simulink model "DR18E_Testpult"  (R2017a)
settings: Solver=ode1  StartTime=0.0  StopTime=Inf  FixedStep=0.001  RelTol=1e-3
PostLoadFcn:
  | , if any(exist('dsrtsu_mdlpostloadfcn', 'file') == [2, 3, 6]), try dsrtsu_mdlpostloadfcn('Execute', bdroot); catch fprintf('Error in PostLoadFcn (dsrtsu_mdlpostloadfcn) for model "%s":\n %s\n', bdroot, lasterr); end, end,
model workspace: external: MATLAB File C:\Users\DeltaRacing\Documents\dSPACE\MABX_DR18E\Model\DR18E_MABX_Parameter.m (data not in the file)
values from neighbouring files (symbols this model uses):
  am = 1/Ts    (= 1)    [DR18E_MABX_Parameter.m]
  bm = K/Ts    (= 0.05)    [DR18E_MABX_Parameter.m]
  cf = 41350    [DR18E_MABX_Parameter.m]
  cr = 41350    [DR18E_MABX_Parameter.m]
  Derating_HV_Battery_Kapa = 1    [DR18E_MABX_Parameter.m]
  Derating_Start_km = 16    [DR18E_MABX_Parameter.m]
  Drive_Mode = 0    [DR18E_MABX_Parameter.m]
  g = 1    [DR18E_MABX_Parameter.m]
  Gas_Modus = 2    [DR18E_MABX_Parameter.m]
  HV_Power_max = 80    [DR18E_MABX_Parameter.m]
  i_Getriebe = 3.3    [DR18E_MABX_Parameter.m]
  i_Lenkgetriebe = 4.32    [DR18E_MABX_Parameter.m]
  K_SET = 1    [DR18E_MABX_Parameter.m]
  Kapazitaet_HV_Battery_kWh = 6.6    [DR18E_MABX_Parameter.m]
  KW_T_Soll = 37    [DR18E_MABX_Parameter.m]
  lf = 1.2    [DR18E_MABX_Parameter.m]
  lr = 1.15    [DR18E_MABX_Parameter.m]
  m = 310    [DR18E_MABX_Parameter.m]
  M_max = 150    [DR18E_MABX_Parameter.m]
  Power_Limit_onoff = 0    [DR18E_MABX_Parameter.m]
  Reifenradius = 0.2351    [DR18E_MABX_Parameter.m]
  Strecke_Endu_km = 22    [DR18E_MABX_Parameter.m]
  TC_Decr_Gas = 0.00005    (= 5e-05)    [DR18E_MABX_Parameter.m]
  TC_Derivative = 0.4    [DR18E_MABX_Parameter.m]
  TC_Incr_Gas = 0.005    [DR18E_MABX_Parameter.m]
  TC_On = 0    [DR18E_MABX_Parameter.m]
  TC_Relay_Off = 0.065    [DR18E_MABX_Parameter.m]
  TC_Relay_On = 0.07    [DR18E_MABX_Parameter.m]
  TV_Mode = 2    [DR18E_MABX_Parameter.m]
  TV_On = 0    [DR18E_MABX_Parameter.m]
  TV_Override = 1    [DR18E_MABX_Parameter.m]
  y = 0.8    [DR18E_MABX_Parameter.m]
undefined symbols (not defined in the file or in its folder): D, DiscIntNeverNeededParam, I, K_OL, P
libraries: simulink x288, rtican x105, rtiusbflightreclib x40, rti1401lib_dio_type3 x10, simulink_extras x10, rti1401lib_adc_type4 x8, rti1401lib_II_base x7
(part 18 of 28)

== system DR18E_Testpult/Verarbeitung/DR18E Torque Control/Derating ==
  note: wenn deltaStrecke
      | > 0 kein Derating
      | < 0 Derating
  In1 : Inport
  0-1 : Saturate  UpperLimit=1  LowerLimit=0
  0-80 : Saturate  UpperLimit=80  LowerLimit=0
  Bus Selector : BusSelector  OutputSignals=TagesenergieMABX_Wh,TagesmeterMABX_m
  Bus Selector1 : BusSelector  OutputSignals=TagesenergieMABX_Wh,TagesmeterMABX_m
  Constant2 : Constant  Value=HV_Power_max
  Derating_Strategie_Reichweite : Subsystem
  MinMax : MinMax  Inputs=2
  Product : Product
  PowerLimit_kW : Outport
  wires:
  In1/1 -> Bus Selector1/1, Bus Selector/1
  Bus Selector/1 -> Derating_Strategie_Reichweite/1(In1)  "<TagesenergieMABX_Wh>"
  Bus Selector/2 -> Derating_Strategie_Reichweite/2(In2)  "<TagesmeterMABX_m>"
  Derating_Strategie_Reichweite/1(deltaStrecke_km) -> MinMax/1
  MinMax/1 -> 0-1/1
  Constant2/1 -> 0-80/1
  Product/1 -> PowerLimit_kW/1
  0-1/1 -> Product/2
  0-80/1 -> Product/1

== system DR18E_Testpult/Verarbeitung/DR18E Torque Control/FlightRecorder ==
  In1 : Inport
  Data Type Conversion : DataTypeConversion
  Gain : Gain
  USB_FLIGHT_REC_BL1 : rtiusbflightreclib/USB_FLIGHT_REC_BL1  VarName=M_max_pro_Mot_Nm  DataType=Single  SampleTime=-1  TLCFileName=rtiusbflightrecwrite  Reserved1=[]  Reserved2=[]  Reserved3=[]  Reserved4=[]  DSProperties=struct('RTI',struct('Version',uint32(3),'BlockType',struct('isSLSource',uint8(0),'isSLSink',uint8(1),'isHWSource',uint8(0),'isHWSink',uint8(0),'isSetup',uint8(0),'isInline',uint8(1),'isNonInline',uint8(0),'isInterrupt',uint8(0),'isChannelwise',uint8(0)),'IOBoardType',{{'DSUSB','FLIGHTREC'}},'UnitType','FLIGHTREC','Identifier','WRITE','DialogType','SL','BlockSet','RTIUSBFLIGHTREC','SlaveProcessor','NONE'))  RTIBlockInterface=struct('InputPortsActive',1,'InputPortsWidth',int32(1),'InputPortsDataType',{{'SS_SINGLE'}},'BlockDisplay',{{['Write to\nUSB Flight Recorder'],'center'}},'IconTransparency','off','InitLevel',3,'BlockName',struct('Token',{{'USB_FLIGHT_REC_BL1'}}),'MaskDescription',['Write input to the Flight Recorder. Recorded data can be referenced by the specified variable.'],'SampleTime',{{-1}})  RTIBlockParameters=struct('VarName',{{'M_max_pro_Mot_Nm','OFF',[]}},'DataType',{{'Single','OFF',[]}},'SampleTime',{{-1,'OFF',[]}},'TLCFileName',{{'rtiusbflightrecwrite','OFF',[]}})  RTISFcnParameters=struct('VarName','char','DataType','char','SampleTime','double','TLCFileName','char')  RTIBlockParaDefault=struct('VarName','Var1','DataType','Single','SampleTime',-1,'TLCFileName','rtiusbflightrecwrite')
      settings: SourceProductName=dSPACE RTI USB Flight Rec Blockset
  wires:
  Gain/1 -> Data Type Conversion/1
  In1/1 -> Gain/1
  Data Type Conversion/1 -> USB_FLIGHT_REC_BL1/1

== system DR18E_Testpult/Verarbeitung/DR18E Torque Control/Power Limit ==
  note: M = P / (2*pi*n)
  note: Power Limit Calculation
  Power Limit onoff : Inport
  DriverTorqueRequest L [Nm] : Inport  Port=2
  DriverTorqueRequest R [Nm] : Inport  Port=3
  Inputs : Inport  Port=4
  Power Limit kW : Inport  Port=5
  Bus Selector : BusSelector  OutputSignals=HV_Power_Watt,Bus.Drehzahl_RL_rad/s,Bus.Drehzahl_RR_rad/s
  Demux : Demux  Outputs=2
  Divide : Product  Inputs=*/
  Divide1 : Product  Inputs=*/
  Divide2 : Product  Inputs=*/
  Logical Operator : Logic  Operator=NOT  AllPortsSameDT=off  OutDataTypeStr=boolean
  Logical Operator1 : Logic  Operator=OR  AllPortsSameDT=off  OutDataTypeStr=boolean
  Mux : Mux  Inputs=2
  Mux1 : Mux  Inputs=2
  Power Limit truefalse : RelationalOperator  Operator=<=  RndMeth=Nearest
  PowerLimit [kW]2 : Constant  Value=0.1
  Product : Product
  RPM-1/s : Gain  Gain=2*pi/(60)
  RPM-1/s1 : Gain  Gain=2*pi/(60)
  Sum1 : Sum  Inputs=-|+
  Sum2 : Sum  Inputs=|++
  Sum3 : Sum  Inputs=++|
  Sum5 : Sum  Inputs=++|
  Switch : Switch  Criteria=u2 > Threshold
  eps : Constant  Value=0.1
  halbe Gesamtleistung pro Motor : Gain  Gain=0.5
  kW-W : Gain  Gain=1000
  "rad/s -> RPM" : Gain  Gain=60/2*pi
  "rad/s -> RPM1" : Gain  Gain=60/2*pi
  LimitedTorque L [Nm] : Outport
  LimitedTorque R [Nm] : Outport  Port=2
  wires:
  Bus Selector/1 -> Power Limit truefalse/1  "<HV_Power_Watt>"
  Power Limit kW/1 -> kW-W/1
  DriverTorqueRequest L [Nm]/1 -> Divide/1, Mux/1
  DriverTorqueRequest R [Nm]/1 -> Sum5/1, Mux/2
  Demux/1 -> LimitedTorque L [Nm]/1
  Demux/2 -> LimitedTorque R [Nm]/1
  Divide/1 -> Product/1
  Product/1 -> Divide1/1, Sum1/1  "PMotL"
  halbe Gesamtleistung pro Motor/1 -> Product/2
  Mux1/1 -> Switch/3  "Torque_in_lim"
  Sum1/1 -> Divide2/1  "PMotR"
  Sum3/1 -> RPM-1/s1/1
  Sum2/1 -> RPM-1/s/1
  eps/1 -> Sum3/1, Sum2/2
  RPM-1/s/1 -> Divide1/2
  RPM-1/s1/1 -> Divide2/2
  Bus Selector/3 -> "rad/s -> RPM1"/1  "<Drehzahl_RR_rad/s>"
  "rad/s -> RPM"/1 -> Sum2/1
  "rad/s -> RPM1"/1 -> Sum3/2
  Divide2/1 -> Mux1/2  "MR"
  Divide1/1 -> Mux1/1  "ML"
  PowerLimit [kW]2/1 -> Sum5/2
  Sum5/1 -> Divide/2
  kW-W/1 -> Sum1/2, Power Limit truefalse/2, halbe Gesamtleistung pro Motor/1
  Power Limit truefalse/1 -> Logical Operator1/2  "Input_Threshold"
  Inputs/1 -> Bus Selector/1
  Bus Selector/2 -> "rad/s -> RPM"/1  "<Drehzahl_RL_rad/s>"
  Switch/1 -> Demux/1  "Torque_out"
  Mux/1 -> Switch/1  "Torque_in"
  Logical Operator/1 -> Logical Operator1/1
  Power Limit onoff/1 -> Logical Operator/1
  Logical Operator1/1 -> Switch/2  "Power Limit aktivnaktiv"

== system DR18E_Testpult/Verarbeitung/DR18E Torque Control/TC RL ==
  TC_On : Inport
  Gas_0-1 : Inport  Port=2
  Inputs : Inport  Port=3
  Bus Selector : BusSelector  OutputSignals=long_slip_left
  Switch : Switch  Criteria=u2 > Threshold
  Traction Control RL : Subsystem
  Logs : Outport
  Motor_Gas_RL : Outport  Port=2
  wires:
  Bus Selector/1 -> Traction Control RL/2(Car.LongSlip)  "<long_slip_left>"
  Gas_0-1/1 -> Switch/3, Traction Control RL/1(Gas_0-1)
  Switch/1 -> Motor_Gas_RL/1
  TC_On/1 -> Switch/2
  Traction Control RL/1(E_Gas) -> Logs/1, Switch/1  "E_Gas_RL"
  Inputs/1 -> Bus Selector/1

== system DR18E_Testpult/Verarbeitung/DR18E Torque Control/TC RR ==
  TC_On : Inport
  Gas_0-1 : Inport  Port=2
  Inputs : Inport  Port=3
  Bus Selector : BusSelector  OutputSignals=long_slip_right
  Switch : Switch  Criteria=u2 > Threshold
  Traction Control RR : Subsystem
  Logs : Outport
  Motor_Gas_RR : Outport  Port=2
  wires:
  Bus Selector/1 -> Traction Control RR/2(Car.LongSlip)  "<long_slip_right>"
  Gas_0-1/1 -> Switch/3, Traction Control RR/1(Gas_0-1)
  Switch/1 -> Motor_Gas_RR/1
  TC_On/1 -> Switch/2
  Traction Control RR/1(E_Gas) -> Logs/1, Switch/1  "E_Gas_RR"
  Inputs/1 -> Bus Selector/1

== system DR18E_Testpult/Verarbeitung/DR18E Torque Control/TV RL ==
  Inputs : Inport
  Bus Selector : BusSelector  OutputSignals=v_kmh,Bus.signal3.RX_Gyro_deg/s.Yaw_Z,Bus.signal3.RX_Lenkwinkel.Steering
  Bus Selector1 : BusSelector  OutputSignals=Bus.signal3.RX_Lenkwinkel.RX Timeout Error,Bus.signal3.RX_Gyro_deg/s.RX Timeout Error
  Constant1 : Constant  Value=0
  Constant2 : Constant  Value=TV_Mode
  Constant3 : Constant  Value=0
  Constant4 : Constant  Value=TV_On
  Gravity2 : Gain  Gain=K_SET
  Lenkwinkel-->Radeinschlagwinkel : Gain  Gain=1/i_Lenkgetriebe
  Logical Operator1 : Logic  AllPortsSameDT=off  OutDataTypeStr=boolean
  MRAC_PT1_Lyapunov : Subsystem
  MRAC_PT1_MIT_DIFF : Subsystem
  MRAC_PT1_MIT_NORM : Subsystem
  Multiport Switch TV : MultiPortSwitch  Inputs=5  DataPortForDefault=Additional data port
  Safety TV off : Logic  Operator=NOR  AllPortsSameDT=off  OutDataTypeStr=boolean
  Switch : Switch  Criteria=u2 > Threshold
  TV DR17E : Subsystem
  TV IPG : Subsystem
  "YawRate SET_NEW " : Subsystem
  deg-rad : Gain  Gain=2*pi/360
  deg-rad1 : Gain  Gain=2*pi/360
  kmh-ms : Gain  Gain=1/3.6
  TV RL Nm : Outport
  wires:
  Inputs/1 -> Bus Selector1/1, Bus Selector/1
  Gravity2/1 -> MRAC_PT1_Lyapunov/1(YawRate REF (rad/s)), MRAC_PT1_MIT_DIFF/1(YawRate REF (rad/s)), MRAC_PT1_MIT_NORM/1(YawRate REF (rad/s))
  "YawRate SET_NEW "/1(YawRate REF (rad/s)) -> Gravity2/1
  TV IPG/1(Out1) -> Multiport Switch TV/2
  MRAC_PT1_Lyapunov/1(Delta M (Nm)) -> Multiport Switch TV/3
  MRAC_PT1_MIT_NORM/1(Delta M (Nm)) -> Multiport Switch TV/4
  MRAC_PT1_MIT_DIFF/1(Delta M (Nm)) -> Multiport Switch TV/5
  Switch/1 -> TV RL Nm/1
  Multiport Switch TV/1 -> Switch/1  "Delta M Nm"
  Constant1/1 -> Switch/3
  Constant2/1 -> Multiport Switch TV/1
  Constant3/1 -> Multiport Switch TV/7
  Bus Selector1/1 -> Safety TV off/1  "<RX Timeout Error>"
  TV DR17E/1(Delta M (Nm)) -> Multiport Switch TV/6
  Constant4/1 -> Logical Operator1/1
  Logical Operator1/1 -> Switch/2
  Safety TV off/1 -> Logical Operator1/2
  Bus Selector/1 -> kmh-ms/1  "<v_kmh>"
  Bus Selector/2 -> TV DR17E/3(psipunkt_ist_deg_s), deg-rad/1  "<Yaw_Z>"
  deg-rad/1 -> MRAC_PT1_MIT_DIFF/2(Car.YawRate), MRAC_PT1_MIT_NORM/2(Car.YawRate), MRAC_PT1_Lyapunov/2(Car.YawRate), TV IPG/2(In3)
  Lenkwinkel-->Radeinschlagwinkel/1 -> TV DR17E/2(Radeinschlagwinkel_deg), deg-rad1/1
  kmh-ms/1 -> TV DR17E/1(vx_ms), "YawRate SET_NEW "/2(v_ms), TV IPG/1(In2)
  Bus Selector/3 -> Lenkwinkel-->Radeinschlagwinkel/1  "<Steering>"
  deg-rad1/1 -> "YawRate SET_NEW "/1(Radeinschlagwinkel_rad)
  Bus Selector1/2 -> Safety TV off/2  "<RX Timeout Error>"

== system DR18E_Testpult/Verarbeitung/DR18E Torque Control/TV RR ==
  Inputs : Inport
  Bus Selector : BusSelector  OutputSignals=v_kmh,Bus.signal3.RX_Gyro_deg/s.Yaw_Z,Bus.signal3.RX_Lenkwinkel.Steering
  Bus Selector1 : BusSelector  OutputSignals=Bus.signal3.RX_Gyro_deg/s.RX Timeout Error,Bus.signal3.RX_Lenkwinkel.RX Timeout Error
  Constant1 : Constant  Value=0
  Constant2 : Constant  Value=TV_Mode
  Constant3 : Constant  Value=0
  Constant4 : Constant  Value=TV_On
  Gravity2 : Gain  Gain=K_SET
  Lenkwinkel-->Radeinschlagwinkel : Gain  Gain=1/i_Lenkgetriebe
  Logical Operator1 : Logic  AllPortsSameDT=off  OutDataTypeStr=boolean
  MRAC_PT1_Lyapunov : Subsystem
  MRAC_PT1_MIT_DIFF : Subsystem
  MRAC_PT1_MIT_NORM : Subsystem
  Multiport Switch TV : MultiPortSwitch  Inputs=5  DataPortForDefault=Additional data port
  Safety TV off : Logic  Operator=NOR  AllPortsSameDT=off  OutDataTypeStr=boolean
  Switch : Switch  Criteria=u2 > Threshold
  TV DR17E : Subsystem
  TV IPG : Subsystem
  "YawRate SET_NEW " : Subsystem
  deg-rad : Gain  Gain=2*pi/360
  deg-rad1 : Gain  Gain=2*pi/360
  kmh-ms : Gain  Gain=1/3.6
  TV RR Nm : Outport
  wires:
  Inputs/1 -> Bus Selector1/1, Bus Selector/1
  Gravity2/1 -> MRAC_PT1_Lyapunov/1(YawRate REF (rad/s)), MRAC_PT1_MIT_DIFF/1(YawRate REF (rad/s)), MRAC_PT1_MIT_NORM/1(YawRate REF (rad/s))
  "YawRate SET_NEW "/1(YawRate REF (rad/s)) -> Gravity2/1
  TV IPG/1(Out1) -> Multiport Switch TV/2
  MRAC_PT1_Lyapunov/1(Delta M (Nm)) -> Multiport Switch TV/3
  MRAC_PT1_MIT_NORM/1(Delta M (Nm)) -> Multiport Switch TV/4
  MRAC_PT1_MIT_DIFF/1(Delta M (Nm)) -> Multiport Switch TV/5
  Switch/1 -> TV RR Nm/1
  Multiport Switch TV/1 -> Switch/1  "Delta M Nm"
  Constant1/1 -> Switch/3
  Constant2/1 -> Multiport Switch TV/1
  Constant3/1 -> Multiport Switch TV/7
  Bus Selector1/1 -> Safety TV off/1  "<RX Timeout Error>"
  TV DR17E/1(Delta M (Nm)) -> Multiport Switch TV/6
  Constant4/1 -> Logical Operator1/1
  Logical Operator1/1 -> Switch/2
  Safety TV off/1 -> Logical Operator1/2
  Bus Selector/1 -> kmh-ms/1  "<v_kmh>"
  Bus Selector/2 -> TV DR17E/3(psipunkt_ist_deg_s), deg-rad/1  "<Yaw_Z>"
  deg-rad/1 -> MRAC_PT1_MIT_DIFF/2(Car.YawRate), MRAC_PT1_MIT_NORM/2(Car.YawRate), MRAC_PT1_Lyapunov/2(Car.YawRate), TV IPG/2(In3)
  Lenkwinkel-->Radeinschlagwinkel/1 -> TV DR17E/2(Radeinschlagwinkel_deg), deg-rad1/1
  kmh-ms/1 -> TV DR17E/1(vx_ms), "YawRate SET_NEW "/2(v_ms), TV IPG/1(In2)
  Bus Selector/3 -> Lenkwinkel-->Radeinschlagwinkel/1  "<Steering>"
  deg-rad1/1 -> "YawRate SET_NEW "/1(Radeinschlagwinkel_rad)
  Bus Selector1/2 -> Safety TV off/2  "<RX Timeout Error>"

== system DR18E_Testpult/Verarbeitung/DR18E Torque Control/Torque Filter ==
  TorqueIn : Inport
  Constant1 : Constant
  Constant2 : Constant
  Demux : Demux  Outputs=2
  Detect Decrease : simulink/Logic and Bit Operations/Detect Decrease  vinit=0.0  InputProcessing=Inherited  OutDataTypeStr=boolean
  Detect Decrease1 : simulink/Logic and Bit Operations/Detect Decrease  vinit=0.0  InputProcessing=Inherited  OutDataTypeStr=boolean
  Detect Increase : simulink/Logic and Bit Operations/Detect Increase  vinit=0.0  InputProcessing=Inherited  OutDataTypeStr=boolean
  Detect Increase1 : simulink/Logic and Bit Operations/Detect Increase  vinit=0.0  InputProcessing=Inherited  OutDataTypeStr=boolean
  M_max : Constant  Value=M_max
  MinTorque : Constant  Value=0
  Mux : Mux  Inputs=2
  PT1 Discrete1 : Subsystem
  PT1 Discrete3 : Subsystem
  S-R Flip-Flop : simulink_extras/Flip Flops/S-R Flip-Flop  initial_condition=0
  S-R Flip-Flop1 : simulink_extras/Flip Flops/S-R Flip-Flop  initial_condition=0
  Saturation Dynamic : simulink/Discontinuities/Saturation Dynamic  OutMin=[]  OutMax=[]  OutDataTypeStr=Inherit: Same as second input  OutDataType=fixdt(1, 16)  OutScaling=2^-10  DoSatur=off
  Switch1 : Switch  Criteria=u2 > Threshold
  Switch2 : Switch  Criteria=u2 > Threshold
  TFilterTorqueFall : Constant  Value=0.01
  TFilterTorqueRise : Constant  Value=0.1
  TorqueFilterOut : Outport
  MaxTorqueOut : Outport  Port=2
  wires:
  Constant2/1 -> PT1 Discrete3/2(K)
  Demux/1 -> PT1 Discrete3/1(u), Detect Increase/1, Detect Decrease/1
  TFilterTorqueRise/1 -> Switch2/1, Switch1/1
  Detect Increase/1 -> S-R Flip-Flop/1
  TFilterTorqueFall/1 -> Switch1/3, Switch2/3
  Switch1/1 -> PT1 Discrete3/3(T)
  Detect Decrease/1 -> S-R Flip-Flop/2
  S-R Flip-Flop/1 -> Switch1/2
  PT1 Discrete3/1(y) -> Mux/1
  Constant1/1 -> PT1 Discrete1/2(K)
  Demux/2 -> Detect Decrease1/1, Detect Increase1/1, PT1 Discrete1/1(u)
  Detect Increase1/1 -> S-R Flip-Flop1/1
  Switch2/1 -> PT1 Discrete1/3(T)
  Detect Decrease1/1 -> S-R Flip-Flop1/2
  S-R Flip-Flop1/1 -> Switch2/2
  TorqueIn/1 -> Demux/1
  PT1 Discrete1/1(y) -> Mux/2
  Mux/1 -> Saturation Dynamic/2
  Saturation Dynamic/1 -> TorqueFilterOut/1
  MinTorque/1 -> Saturation Dynamic/3
  M_max/1 -> MaxTorqueOut/1, Saturation Dynamic/1

== system DR18E_Testpult/Verarbeitung/Gaspedal Check/Add_Software_inplausible_Warning ==
  note: Fehlercode AA, wenn Software Inplausibilität erkennt
  Softw_Plausibel : Inport
  Error_Code : Inport  Port=2
  Compare To Zero : simulink/Logic and Bit Operations/Compare To Zero  relop===  OutDataTypeStr=boolean
  Constant : Constant  Value=hex2dec('AA')
  Switch : Switch  Criteria=u2 > Threshold
  ErrorCode_Out : Outport
  wires:
  Softw_Plausibel/1 -> Compare To Zero/1
  Error_Code/1 -> Switch/3
  Constant/1 -> Switch/1
  Switch/1 -> ErrorCode_Out/1
  Compare To Zero/1 -> Switch/2

== system DR18E_Testpult/Verarbeitung/Gaspedal Check/Add_Software_inplausible_Warning1 ==
  note: Fehlercode AA, wenn Software Inplausibilität erkennt
  Softw_Plausibel : Inport
  Error_Code : Inport  Port=2
  Compare To Zero : simulink/Logic and Bit Operations/Compare To Zero  relop===  OutDataTypeStr=boolean
  Constant : Constant  Value=hex2dec('AA')
  Switch : Switch  Criteria=u2 > Threshold
  ErrorCode_Out : Outport
  wires:
  Softw_Plausibel/1 -> Compare To Zero/1
  Error_Code/1 -> Switch/3
  Constant/1 -> Switch/1
  Switch/1 -> ErrorCode_Out/1
  Compare To Zero/1 -> Switch/2

== system DR18E_Testpult/Verarbeitung/Gaspedal Check/FlightRecorder ==
  In1 : Inport
  Data Type Conversion : DataTypeConversion
  Gain : Gain  Gain=100
  USB_FLIGHT_REC_BL1 : rtiusbflightreclib/USB_FLIGHT_REC_BL1  VarName=gas_plausibel_prozent  DataType=Single  SampleTime=-1  TLCFileName=rtiusbflightrecwrite  Reserved1=[]  Reserved2=[]  Reserved3=[]  Reserved4=[]  DSProperties=struct('RTI',struct('Version',uint32(3),'BlockType',struct('isSLSource',uint8(0),'isSLSink',uint8(1),'isHWSource',uint8(0),'isHWSink',uint8(0),'isSetup',uint8(0),'isInline',uint8(1),'isNonInline',uint8(0),'isInterrupt',uint8(0),'isChannelwise',uint8(0)),'IOBoardType',{{'DSUSB','FLIGHTREC'}},'UnitType','FLIGHTREC','Identifier','WRITE','DialogType','SL','BlockSet','RTIUSBFLIGHTREC','SlaveProcessor','NONE'))  RTIBlockInterface=struct('InputPortsActive',1,'InputPortsWidth',int32(1),'InputPortsDataType',{{'SS_SINGLE'}},'BlockDisplay',{{['Write to\nUSB Flight Recorder'],'center'}},'IconTransparency','off','InitLevel',3,'BlockName',struct('Token',{{'USB_FLIGHT_REC_BL1'}}),'MaskDescription',['Write input to the Flight Recorder. Recorded data can be referenced by the specified variable.'],'SampleTime',{{-1}})  RTIBlockParameters=struct('VarName',{{'gas_plausibel_prozent','OFF',[]}},'DataType',{{'Single','OFF',[]}},'SampleTime',{{-1,'OFF',[]}},'TLCFileName',{{'rtiusbflightrecwrite','OFF',[]}})  RTISFcnParameters=struct('VarName','char','DataType','char','SampleTime','double','TLCFileName','char')  RTIBlockParaDefault=struct('VarName','Var1','DataType','Single','SampleTime',-1,'TLCFileName','rtiusbflightrecwrite')
      settings: SourceProductName=dSPACE RTI USB Flight Rec Blockset
  wires:
  Data Type Conversion/1 -> USB_FLIGHT_REC_BL1/1
  In1/1 -> Gain/1
  Gain/1 -> Data Type Conversion/1

== system DR18E_Testpult/Verarbeitung/Gaspedal Check/PlausibilityCheck ==
  note: Output is zero,
      | if Inplausibility is detected
  note: use filtered Signals for Plausibility Check
  note: Always pass through lower value,
      | if signal is plausible
  Gas1 : Inport
  Gas2 : Inport  Port=2
  Abs1 : Abs
  Constant : Constant  Value=0
  Constant1 : Constant
  Constant2 : Constant
  Constant3 : Constant  Value=2
  Divide : Product  Inputs=*/
  Gain : Gain  Gain=1/100
  Min : MinMax  Inputs=2
  PT1 Discrete : Subsystem
  PT1 Discrete1 : Subsystem
  Rule: T10.3.9 : simulink/Logic and Bit Operations/Compare To Constant  relop=>  const=10  OutDataTypeStr=boolean
  Saturation : Saturate  UpperLimit=100  LowerLimit=0
  Saturation1 : Saturate  UpperLimit=100  LowerLimit=0
  Sum : Sum  Inputs=|+-
  Sum1 : Sum  Inputs=|++
  Switch : Switch  Criteria=u2 > Threshold
  TFilterGas1 : Constant  Value=0.1
  TFilterGas2 : Constant  Value=0.1
  Gas_0-1_plausibel : Outport
  wires:
  Sum/1 -> Abs1/1
  PT1 Discrete1/1(y) -> Sum/2
  PT1 Discrete/1(y) -> Sum/1
  Rule: T10.3.9/1 -> Switch/2  "Plausibel"
  Constant/1 -> Switch/1
  Switch/1 -> Gas_0-1_plausibel/1
  Constant1/1 -> PT1 Discrete/2(K)
  TFilterGas1/1 -> PT1 Discrete/3(T)
  Gas1/1 -> Saturation/1
  Constant2/1 -> PT1 Discrete1/2(K)
  TFilterGas2/1 -> PT1 Discrete1/3(T)
  Gas2/1 -> Saturation1/1
  Saturation/1 -> Sum1/1, PT1 Discrete/1(u)
  Saturation1/1 -> Sum1/2, PT1 Discrete1/1(u)
  Abs1/1 -> Rule: T10.3.9/1  "PlausAbs"
  Divide/1 -> Gain/1  "ThrottleMean"
  Sum1/1 -> Divide/1
  Constant3/1 -> Divide/2
  Gain/1 -> Switch/3

== system DR18E_Testpult/Verarbeitung/Gaspedal Check/Testmodus ==
  Gas1 : Inport
  Gas2 : Inport  Port=2
  Gain : Gain  Gain=1/100
  Gas_manuell_0100 : Constant  Value=0
  Gas_manuell_2off1on : Constant  Value=2
  Min : MinMax  Function=max  Inputs=2
  Multiport Switch : MultiPortSwitch  Inputs=2
  Saturation : Saturate  UpperLimit=100  LowerLimit=0
  Saturation1 : Saturate  UpperLimit=100  LowerLimit=0
  Saturation2 : Saturate  UpperLimit=100  LowerLimit=0
  Gas_0-1 : Outport
  wires:
  Gain/1 -> Gas_0-1/1
  Gas1/1 -> Saturation/1
  Gas2/1 -> Saturation1/1
  Saturation/1 -> Min/1
  Saturation1/1 -> Min/2
  Gas_manuell_0100/1 -> Saturation2/1
  Saturation2/1 -> Multiport Switch/2
  Min/1 -> Multiport Switch/3
  Multiport Switch/1 -> Gain/1
  Gas_manuell_2off1on/1 -> Multiport Switch/1

== system DR18E_Testpult/Verarbeitung/MABX RAM/FlightRecorder5 ==
  In1 : Inport
  Data Type Conversion : DataTypeConversion
  Gain : Gain
  USB_FLIGHT_REC_BL1 : rtiusbflightreclib/USB_FLIGHT_REC_BL1  VarName=gesamt_s_m  DataType=Single  SampleTime=-1  TLCFileName=rtiusbflightrecwrite  Reserved1=[]  Reserved2=[]  Reserved3=[]  Reserved4=[]  DSProperties=struct('RTI',struct('Version',uint32(3),'BlockType',struct('isSLSource',uint8(0),'isSLSink',uint8(1),'isHWSource',uint8(0),'isHWSink',uint8(0),'isSetup',uint8(0),'isInline',uint8(1),'isNonInline',uint8(0),'isInterrupt',uint8(0),'isChannelwise',uint8(0)),'IOBoardType',{{'DSUSB','FLIGHTREC'}},'UnitType','FLIGHTREC','Identifier','WRITE','DialogType','SL','BlockSet','RTIUSBFLIGHTREC','SlaveProcessor','NONE'))  RTIBlockInterface=struct('InputPortsActive',1,'InputPortsWidth',int32(1),'InputPortsDataType',{{'SS_SINGLE'}},'BlockDisplay',{{['Write to\nUSB Flight Recorder'],'center'}},'IconTransparency','off','InitLevel',3,'BlockName',struct('Token',{{'USB_FLIGHT_REC_BL1'}}),'MaskDescription',['Write input to the Flight Recorder. Recorded data can be referenced by the specified variable.'],'SampleTime',{{-1}})  RTIBlockParameters=struct('VarName',{{'gesamt_s_m','OFF',[]}},'DataType',{{'Single','OFF',[]}},'SampleTime',{{-1,'OFF',[]}},'TLCFileName',{{'rtiusbflightrecwrite','OFF',[]}})  RTISFcnParameters=struct('VarName','char','DataType','char','SampleTime','double','TLCFileName','char')  RTIBlockParaDefault=struct('VarName','Var1','DataType','Single','SampleTime',-1,'TLCFileName','rtiusbflightrecwrite')
      settings: SourceProductName=dSPACE RTI USB Flight Rec Blockset
  wires:
  Data Type Conversion/1 -> USB_FLIGHT_REC_BL1/1
  In1/1 -> Gain/1
  Gain/1 -> Data Type Conversion/1

== system DR18E_Testpult/Verarbeitung/Precalculations/FlightRecorder ==
  In1 : Inport
  Data Type Conversion : DataTypeConversion
  Gain : Gain
  USB_FLIGHT_REC_BL1 : rtiusbflightreclib/USB_FLIGHT_REC_BL1  VarName=v_kmh  DataType=Single  SampleTime=-1  TLCFileName=rtiusbflightrecwrite  Reserved1=[]  Reserved2=[]  Reserved3=[]  Reserved4=[]  DSProperties=struct('RTI',struct('Version',uint32(3),'BlockType',struct('isSLSource',uint8(0),'isSLSink',uint8(1),'isHWSource',uint8(0),'isHWSink',uint8(0),'isSetup',uint8(0),'isInline',uint8(1),'isNonInline',uint8(0),'isInterrupt',uint8(0),'isChannelwise',uint8(0)),'IOBoardType',{{'DSUSB','FLIGHTREC'}},'UnitType','FLIGHTREC','Identifier','WRITE','DialogType','SL','BlockSet','RTIUSBFLIGHTREC','SlaveProcessor','NONE'))  RTIBlockInterface=struct('InputPortsActive',1,'InputPortsWidth',int32(1),'InputPortsDataType',{{'SS_SINGLE'}},'BlockDisplay',{{['Write to\nUSB Flight Recorder'],'center'}},'IconTransparency','off','InitLevel',3,'BlockName',struct('Token',{{'USB_FLIGHT_REC_BL1'}}),'MaskDescription',['Write input to the Flight Recorder. Recorded data can be referenced by the specified variable.'],'SampleTime',{{-1}})  RTIBlockParameters=struct('VarName',{{'v_kmh','OFF',[]}},'DataType',{{'Single','OFF',[]}},'SampleTime',{{-1,'OFF',[]}},'TLCFileName',{{'rtiusbflightrecwrite','OFF',[]}})  RTISFcnParameters=struct('VarName','char','DataType','char','SampleTime','double','TLCFileName','char')  RTIBlockParaDefault=struct('VarName','Var1','DataType','Single','SampleTime',-1,'TLCFileName','rtiusbflightrecwrite')
      settings: SourceProductName=dSPACE RTI USB Flight Rec Blockset
  wires:
  Data Type Conversion/1 -> USB_FLIGHT_REC_BL1/1
  In1/1 -> Gain/1
  Gain/1 -> Data Type Conversion/1

== system DR18E_Testpult/Verarbeitung/Precalculations/FlightRecorder1 ==
  In1 : Inport
  Data Type Conversion : DataTypeConversion
  Gain : Gain
  USB_FLIGHT_REC_BL1 : rtiusbflightreclib/USB_FLIGHT_REC_BL1  VarName=DrehzahlRL_rpm  DataType=Single  SampleTime=-1  TLCFileName=rtiusbflightrecwrite  Reserved1=[]  Reserved2=[]  Reserved3=[]  Reserved4=[]  DSProperties=struct('RTI',struct('Version',uint32(3),'BlockType',struct('isSLSource',uint8(0),'isSLSink',uint8(1),'isHWSource',uint8(0),'isHWSink',uint8(0),'isSetup',uint8(0),'isInline',uint8(1),'isNonInline',uint8(0),'isInterrupt',uint8(0),'isChannelwise',uint8(0)),'IOBoardType',{{'DSUSB','FLIGHTREC'}},'UnitType','FLIGHTREC','Identifier','WRITE','DialogType','SL','BlockSet','RTIUSBFLIGHTREC','SlaveProcessor','NONE'))  RTIBlockInterface=struct('InputPortsActive',1,'InputPortsWidth',int32(1),'InputPortsDataType',{{'SS_SINGLE'}},'BlockDisplay',{{['Write to\nUSB Flight Recorder'],'center'}},'IconTransparency','off','InitLevel',3,'BlockName',struct('Token',{{'USB_FLIGHT_REC_BL1'}}),'MaskDescription',['Write input to the Flight Recorder. Recorded data can be referenced by the specified variable.'],'SampleTime',{{-1}})  RTIBlockParameters=struct('VarName',{{'DrehzahlRL_rpm','OFF',[]}},'DataType',{{'Single','OFF',[]}},'SampleTime',{{-1,'OFF',[]}},'TLCFileName',{{'rtiusbflightrecwrite','OFF',[]}})  RTISFcnParameters=struct('VarName','char','DataType','char','SampleTime','double','TLCFileName','char')  RTIBlockParaDefault=struct('VarName','Var1','DataType','Single','SampleTime',-1,'TLCFileName','rtiusbflightrecwrite')
      settings: SourceProductName=dSPACE RTI USB Flight Rec Blockset
  wires:
  Data Type Conversion/1 -> USB_FLIGHT_REC_BL1/1
  In1/1 -> Gain/1
  Gain/1 -> Data Type Conversion/1

== system DR18E_Testpult/Verarbeitung/Precalculations/FlightRecorder2 ==
  In1 : Inport
  Data Type Conversion : DataTypeConversion
  Gain : Gain
  USB_FLIGHT_REC_BL1 : rtiusbflightreclib/USB_FLIGHT_REC_BL1  VarName=DrehzahlRR_rpm  DataType=Single  SampleTime=-1  TLCFileName=rtiusbflightrecwrite  Reserved1=[]  Reserved2=[]  Reserved3=[]  Reserved4=[]  DSProperties=struct('RTI',struct('Version',uint32(3),'BlockType',struct('isSLSource',uint8(0),'isSLSink',uint8(1),'isHWSource',uint8(0),'isHWSink',uint8(0),'isSetup',uint8(0),'isInline',uint8(1),'isNonInline',uint8(0),'isInterrupt',uint8(0),'isChannelwise',uint8(0)),'IOBoardType',{{'DSUSB','FLIGHTREC'}},'UnitType','FLIGHTREC','Identifier','WRITE','DialogType','SL','BlockSet','RTIUSBFLIGHTREC','SlaveProcessor','NONE'))  RTIBlockInterface=struct('InputPortsActive',1,'InputPortsWidth',int32(1),'InputPortsDataType',{{'SS_SINGLE'}},'BlockDisplay',{{['Write to\nUSB Flight Recorder'],'center'}},'IconTransparency','off','InitLevel',3,'BlockName',struct('Token',{{'USB_FLIGHT_REC_BL1'}}),'MaskDescription',['Write input to the Flight Recorder. Recorded data can be referenced by the specified variable.'],'SampleTime',{{-1}})  RTIBlockParameters=struct('VarName',{{'DrehzahlRR_rpm','OFF',[]}},'DataType',{{'Single','OFF',[]}},'SampleTime',{{-1,'OFF',[]}},'TLCFileName',{{'rtiusbflightrecwrite','OFF',[]}})  RTISFcnParameters=struct('VarName','char','DataType','char','SampleTime','double','TLCFileName','char')  RTIBlockParaDefault=struct('VarName','Var1','DataType','Single','SampleTime',-1,'TLCFileName','rtiusbflightrecwrite')
      settings: SourceProductName=dSPACE RTI USB Flight Rec Blockset
  wires:
  Data Type Conversion/1 -> USB_FLIGHT_REC_BL1/1
  In1/1 -> Gain/1
  Gain/1 -> Data Type Conversion/1

== system DR18E_Testpult/Verarbeitung/Precalculations/FlightRecorder3 ==
  In1 : Inport
  Data Type Conversion : DataTypeConversion
  Gain : Gain
  USB_FLIGHT_REC_BL1 : rtiusbflightreclib/USB_FLIGHT_REC_BL1  VarName=DrehzahlFR_rpm  DataType=Single  SampleTime=-1  TLCFileName=rtiusbflightrecwrite  Reserved1=[]  Reserved2=[]  Reserved3=[]  Reserved4=[]  DSProperties=struct('RTI',struct('Version',uint32(3),'BlockType',struct('isSLSource',uint8(0),'isSLSink',uint8(1),'isHWSource',uint8(0),'isHWSink',uint8(0),'isSetup',uint8(0),'isInline',uint8(1),'isNonInline',uint8(0),'isInterrupt',uint8(0),'isChannelwise',uint8(0)),'IOBoardType',{{'DSUSB','FLIGHTREC'}},'UnitType','FLIGHTREC','Identifier','WRITE','DialogType','SL','BlockSet','RTIUSBFLIGHTREC','SlaveProcessor','NONE'))  RTIBlockInterface=struct('InputPortsActive',1,'InputPortsWidth',int32(1),'InputPortsDataType',{{'SS_SINGLE'}},'BlockDisplay',{{['Write to\nUSB Flight Recorder'],'center'}},'IconTransparency','off','InitLevel',3,'BlockName',struct('Token',{{'USB_FLIGHT_REC_BL1'}}),'MaskDescription',['Write input to the Flight Recorder. Recorded data can be referenced by the specified variable.'],'SampleTime',{{-1}})  RTIBlockParameters=struct('VarName',{{'DrehzahlFR_rpm','OFF',[]}},'DataType',{{'Single','OFF',[]}},'SampleTime',{{-1,'OFF',[]}},'TLCFileName',{{'rtiusbflightrecwrite','OFF',[]}})  RTISFcnParameters=struct('VarName','char','DataType','char','SampleTime','double','TLCFileName','char')  RTIBlockParaDefault=struct('VarName','Var1','DataType','Single','SampleTime',-1,'TLCFileName','rtiusbflightrecwrite')
      settings: SourceProductName=dSPACE RTI USB Flight Rec Blockset
  wires:
  Data Type Conversion/1 -> USB_FLIGHT_REC_BL1/1
  In1/1 -> Gain/1
  Gain/1 -> Data Type Conversion/1

== system DR18E_Testpult/Verarbeitung/Precalculations/FlightRecorder4 ==
  In1 : Inport
  Data Type Conversion : DataTypeConversion
  Gain : Gain
  USB_FLIGHT_REC_BL1 : rtiusbflightreclib/USB_FLIGHT_REC_BL1  VarName=DrehzahlFL_rpm  DataType=Single  SampleTime=-1  TLCFileName=rtiusbflightrecwrite  Reserved1=[]  Reserved2=[]  Reserved3=[]  Reserved4=[]  DSProperties=struct('RTI',struct('Version',uint32(3),'BlockType',struct('isSLSource',uint8(0),'isSLSink',uint8(1),'isHWSource',uint8(0),'isHWSink',uint8(0),'isSetup',uint8(0),'isInline',uint8(1),'isNonInline',uint8(0),'isInterrupt',uint8(0),'isChannelwise',uint8(0)),'IOBoardType',{{'DSUSB','FLIGHTREC'}},'UnitType','FLIGHTREC','Identifier','WRITE','DialogType','SL','BlockSet','RTIUSBFLIGHTREC','SlaveProcessor','NONE'))  RTIBlockInterface=struct('InputPortsActive',1,'InputPortsWidth',int32(1),'InputPortsDataType',{{'SS_SINGLE'}},'BlockDisplay',{{['Write to\nUSB Flight Recorder'],'center'}},'IconTransparency','off','InitLevel',3,'BlockName',struct('Token',{{'USB_FLIGHT_REC_BL1'}}),'MaskDescription',['Write input to the Flight Recorder. Recorded data can be referenced by the specified variable.'],'SampleTime',{{-1}})  RTIBlockParameters=struct('VarName',{{'DrehzahlFL_rpm','OFF',[]}},'DataType',{{'Single','OFF',[]}},'SampleTime',{{-1,'OFF',[]}},'TLCFileName',{{'rtiusbflightrecwrite','OFF',[]}})  RTISFcnParameters=struct('VarName','char','DataType','char','SampleTime','double','TLCFileName','char')  RTIBlockParaDefault=struct('VarName','Var1','DataType','Single','SampleTime',-1,'TLCFileName','rtiusbflightrecwrite')
      settings: SourceProductName=dSPACE RTI USB Flight Rec Blockset
  wires:
  Data Type Conversion/1 -> USB_FLIGHT_REC_BL1/1
  In1/1 -> Gain/1
  Gain/1 -> Data Type Conversion/1

== system DR18E_Testpult/Verarbeitung/Precalculations/FlightRecorder5 ==
  In1 : Inport
  Data Type Conversion : DataTypeConversion
  Gain : Gain
  USB_FLIGHT_REC_BL1 : rtiusbflightreclib/USB_FLIGHT_REC_BL1  VarName=slip_links_0_1  DataType=Single  SampleTime=-1  TLCFileName=rtiusbflightrecwrite  Reserved1=[]  Reserved2=[]  Reserved3=[]  Reserved4=[]  DSProperties=struct('RTI',struct('Version',uint32(3),'BlockType',struct('isSLSource',uint8(0),'isSLSink',uint8(1),'isHWSource',uint8(0),'isHWSink',uint8(0),'isSetup',uint8(0),'isInline',uint8(1),'isNonInline',uint8(0),'isInterrupt',uint8(0),'isChannelwise',uint8(0)),'IOBoardType',{{'DSUSB','FLIGHTREC'}},'UnitType','FLIGHTREC','Identifier','WRITE','DialogType','SL','BlockSet','RTIUSBFLIGHTREC','SlaveProcessor','NONE'))  RTIBlockInterface=struct('InputPortsActive',1,'InputPortsWidth',int32(1),'InputPortsDataType',{{'SS_SINGLE'}},'BlockDisplay',{{['Write to\nUSB Flight Recorder'],'center'}},'IconTransparency','off','InitLevel',3,'BlockName',struct('Token',{{'USB_FLIGHT_REC_BL1'}}),'MaskDescription',['Write input to the Flight Recorder. Recorded data can be referenced by the specified variable.'],'SampleTime',{{-1}})  RTIBlockParameters=struct('VarName',{{'slip_links_0_1','OFF',[]}},'DataType',{{'Single','OFF',[]}},'SampleTime',{{-1,'OFF',[]}},'TLCFileName',{{'rtiusbflightrecwrite','OFF',[]}})  RTISFcnParameters=struct('VarName','char','DataType','char','SampleTime','double','TLCFileName','char')  RTIBlockParaDefault=struct('VarName','Var1','DataType','Single','SampleTime',-1,'TLCFileName','rtiusbflightrecwrite')
      settings: SourceProductName=dSPACE RTI USB Flight Rec Blockset
  wires:
  Data Type Conversion/1 -> USB_FLIGHT_REC_BL1/1
  In1/1 -> Gain/1
  Gain/1 -> Data Type Conversion/1

== system DR18E_Testpult/Verarbeitung/Precalculations/FlightRecorder6 ==
  In1 : Inport
  Data Type Conversion : DataTypeConversion
  Gain : Gain
  USB_FLIGHT_REC_BL1 : rtiusbflightreclib/USB_FLIGHT_REC_BL1  VarName=slip_rechts_0_1  DataType=Single  SampleTime=-1  TLCFileName=rtiusbflightrecwrite  Reserved1=[]  Reserved2=[]  Reserved3=[]  Reserved4=[]  DSProperties=struct('RTI',struct('Version',uint32(3),'BlockType',struct('isSLSource',uint8(0),'isSLSink',uint8(1),'isHWSource',uint8(0),'isHWSink',uint8(0),'isSetup',uint8(0),'isInline',uint8(1),'isNonInline',uint8(0),'isInterrupt',uint8(0),'isChannelwise',uint8(0)),'IOBoardType',{{'DSUSB','FLIGHTREC'}},'UnitType','FLIGHTREC','Identifier','WRITE','DialogType','SL','BlockSet','RTIUSBFLIGHTREC','SlaveProcessor','NONE'))  RTIBlockInterface=struct('InputPortsActive',1,'InputPortsWidth',int32(1),'InputPortsDataType',{{'SS_SINGLE'}},'BlockDisplay',{{['Write to\nUSB Flight Recorder'],'center'}},'IconTransparency','off','InitLevel',3,'BlockName',struct('Token',{{'USB_FLIGHT_REC_BL1'}}),'MaskDescription',['Write input to the Flight Recorder. Recorded data can be referenced by the specified variable.'],'SampleTime',{{-1}})  RTIBlockParameters=struct('VarName',{{'slip_rechts_0_1','OFF',[]}},'DataType',{{'Single','OFF',[]}},'SampleTime',{{-1,'OFF',[]}},'TLCFileName',{{'rtiusbflightrecwrite','OFF',[]}})  RTISFcnParameters=struct('VarName','char','DataType','char','SampleTime','double','TLCFileName','char')  RTIBlockParaDefault=struct('VarName','Var1','DataType','Single','SampleTime',-1,'TLCFileName','rtiusbflightrecwrite')
      settings: SourceProductName=dSPACE RTI USB Flight Rec Blockset
  wires:
  Data Type Conversion/1 -> USB_FLIGHT_REC_BL1/1
  In1/1 -> Gain/1
  Gain/1 -> Data Type Conversion/1

== system DR18E_Testpult/Verarbeitung/Precalculations/kilometer tracking ==
  v_ms : Inport
  Discrete-Time Integrator : DiscreteIntegrator  SampleTime=-1  ICPrevOutput=DiscIntNeverNeededParam  ICPrevScaledInput=DiscIntNeverNeededParam
  FlightRecorder1 : Subsystem
  s_m : Gain
  tag scope: Tagesmeter_s_m=global
  wires:
  v_ms/1 -> Discrete-Time Integrator/1
  s_m/1 -> [Tagesmeter_s_m], FlightRecorder1/1(In1)  "Tagesmeter_fluechtig_s_m"
  Discrete-Time Integrator/1 -> s_m/1

== system DR18E_Testpult/Verarbeitung/Strom//SOC/HVIRecorder ==
  In1 : Inport
  Data Type Conversion : DataTypeConversion
  Gain : Gain
  USB_FLIGHT_REC_BL1 : rtiusbflightreclib/USB_FLIGHT_REC_BL1  VarName=HV_current_A  DataType=Single  SampleTime=-1  TLCFileName=rtiusbflightrecwrite  Reserved1=[]  Reserved2=[]  Reserved3=[]  Reserved4=[]  DSProperties=struct('RTI',struct('Version',uint32(3),'BlockType',struct('isSLSource',uint8(0),'isSLSink',uint8(1),'isHWSource',uint8(0),'isHWSink',uint8(0),'isSetup',uint8(0),'isInline',uint8(1),'isNonInline',uint8(0),'isInterrupt',uint8(0),'isChannelwise',uint8(0)),'IOBoardType',{{'DSUSB','FLIGHTREC'}},'UnitType','FLIGHTREC','Identifier','WRITE','DialogType','SL','BlockSet','RTIUSBFLIGHTREC','SlaveProcessor','NONE'))  RTIBlockInterface=struct('InputPortsActive',1,'InputPortsWidth',int32(1),'InputPortsDataType',{{'SS_SINGLE'}},'BlockDisplay',{{['Write to\nUSB Flight Recorder'],'center'}},'IconTransparency','off','InitLevel',3,'BlockName',struct('Token',{{'USB_FLIGHT_REC_BL1'}}),'MaskDescription',['Write input to the Flight Recorder. Recorded data can be referenced by the specified variable.'],'SampleTime',{{-1}})  RTIBlockParameters=struct('VarName',{{'HV_current_A','OFF',[]}},'DataType',{{'Single','OFF',[]}},'SampleTime',{{-1,'OFF',[]}},'TLCFileName',{{'rtiusbflightrecwrite','OFF',[]}})  RTISFcnParameters=struct('VarName','char','DataType','char','SampleTime','double','TLCFileName','char')  RTIBlockParaDefault=struct('VarName','Var1','DataType','Single','SampleTime',-1,'TLCFileName','rtiusbflightrecwrite')
      settings: SourceProductName=dSPACE RTI USB Flight Rec Blockset
  wires:
  Data Type Conversion/1 -> USB_FLIGHT_REC_BL1/1
  In1/1 -> Gain/1
  Gain/1 -> Data Type Conversion/1

== system DR18E_Testpult/Verarbeitung/Strom//SOC/HVURecorder ==
  In1 : Inport
  Data Type Conversion : DataTypeConversion
  Gain : Gain
  USB_FLIGHT_REC_BL1 : rtiusbflightreclib/USB_FLIGHT_REC_BL1  VarName=HV_voltage_V  DataType=Single  SampleTime=-1  TLCFileName=rtiusbflightrecwrite  Reserved1=[]  Reserved2=[]  Reserved3=[]  Reserved4=[]  DSProperties=struct('RTI',struct('Version',uint32(3),'BlockType',struct('isSLSource',uint8(0),'isSLSink',uint8(1),'isHWSource',uint8(0),'isHWSink',uint8(0),'isSetup',uint8(0),'isInline',uint8(1),'isNonInline',uint8(0),'isInterrupt',uint8(0),'isChannelwise',uint8(0)),'IOBoardType',{{'DSUSB','FLIGHTREC'}},'UnitType','FLIGHTREC','Identifier','WRITE','DialogType','SL','BlockSet','RTIUSBFLIGHTREC','SlaveProcessor','NONE'))  RTIBlockInterface=struct('InputPortsActive',1,'InputPortsWidth',int32(1),'InputPortsDataType',{{'SS_SINGLE'}},'BlockDisplay',{{['Write to\nUSB Flight Recorder'],'center'}},'IconTransparency','off','InitLevel',3,'BlockName',struct('Token',{{'USB_FLIGHT_REC_BL1'}}),'MaskDescription',['Write input to the Flight Recorder. Recorded data can be referenced by the specified variable.'],'SampleTime',{{-1}})  RTIBlockParameters=struct('VarName',{{'HV_voltage_V','OFF',[]}},'DataType',{{'Single','OFF',[]}},'SampleTime',{{-1,'OFF',[]}},'TLCFileName',{{'rtiusbflightrecwrite','OFF',[]}})  RTISFcnParameters=struct('VarName','char','DataType','char','SampleTime','double','TLCFileName','char')  RTIBlockParaDefault=struct('VarName','Var1','DataType','Single','SampleTime',-1,'TLCFileName','rtiusbflightrecwrite')
      settings: SourceProductName=dSPACE RTI USB Flight Rec Blockset
  wires:
  Data Type Conversion/1 -> USB_FLIGHT_REC_BL1/1
  In1/1 -> Gain/1
  Gain/1 -> Data Type Conversion/1

== system DR18E_Testpult/Verarbeitung/Strom//SOC/currentConsumptionRecorder ==
  In1 : Inport
  Data Type Conversion : DataTypeConversion
  Gain : Gain
  USB_FLIGHT_REC_BL1 : rtiusbflightreclib/USB_FLIGHT_REC_BL1  VarName=currentConsumption_As  DataType=Single  SampleTime=-1  TLCFileName=rtiusbflightrecwrite  Reserved1=[]  Reserved2=[]  Reserved3=[]  Reserved4=[]  DSProperties=struct('RTI',struct('Version',uint32(3),'BlockType',struct('isSLSource',uint8(0),'isSLSink',uint8(1),'isHWSource',uint8(0),'isHWSink',uint8(0),'isSetup',uint8(0),'isInline',uint8(1),'isNonInline',uint8(0),'isInterrupt',uint8(0),'isChannelwise',uint8(0)),'IOBoardType',{{'DSUSB','FLIGHTREC'}},'UnitType','FLIGHTREC','Identifier','WRITE','DialogType','SL','BlockSet','RTIUSBFLIGHTREC','SlaveProcessor','NONE'))  RTIBlockInterface=struct('InputPortsActive',1,'InputPortsWidth',int32(1),'InputPortsDataType',{{'SS_SINGLE'}},'BlockDisplay',{{['Write to\nUSB Flight Recorder'],'center'}},'IconTransparency','off','InitLevel',3,'BlockName',struct('Token',{{'USB_FLIGHT_REC_BL1'}}),'MaskDescription',['Write input to the Flight Recorder. Recorded data can be referenced by the specified variable.'],'SampleTime',{{-1}})  RTIBlockParameters=struct('VarName',{{'currentConsumption_As','OFF',[]}},'DataType',{{'Single','OFF',[]}},'SampleTime',{{-1,'OFF',[]}},'TLCFileName',{{'rtiusbflightrecwrite','OFF',[]}})  RTISFcnParameters=struct('VarName','char','DataType','char','SampleTime','double','TLCFileName','char')  RTIBlockParaDefault=struct('VarName','Var1','DataType','Single','SampleTime',-1,'TLCFileName','rtiusbflightrecwrite')
      settings: SourceProductName=dSPACE RTI USB Flight Rec Blockset
  wires:
  Data Type Conversion/1 -> USB_FLIGHT_REC_BL1/1
  In1/1 -> Gain/1
  Gain/1 -> Data Type Conversion/1

== system DR18E_Testpult/Verarbeitung/Strom//SOC/powerConsumtionRecorder ==
  In1 : Inport
  Data Type Conversion : DataTypeConversion
  Gain : Gain
  USB_FLIGHT_REC_BL1 : rtiusbflightreclib/USB_FLIGHT_REC_BL1  VarName=powerConsumption_Ws  DataType=Single  SampleTime=-1  TLCFileName=rtiusbflightrecwrite  Reserved1=[]  Reserved2=[]  Reserved3=[]  Reserved4=[]  DSProperties=struct('RTI',struct('Version',uint32(3),'BlockType',struct('isSLSource',uint8(0),'isSLSink',uint8(1),'isHWSource',uint8(0),'isHWSink',uint8(0),'isSetup',uint8(0),'isInline',uint8(1),'isNonInline',uint8(0),'isInterrupt',uint8(0),'isChannelwise',uint8(0)),'IOBoardType',{{'DSUSB','FLIGHTREC'}},'UnitType','FLIGHTREC','Identifier','WRITE','DialogType','SL','BlockSet','RTIUSBFLIGHTREC','SlaveProcessor','NONE'))  RTIBlockInterface=struct('InputPortsActive',1,'InputPortsWidth',int32(1),'InputPortsDataType',{{'SS_SINGLE'}},'BlockDisplay',{{['Write to\nUSB Flight Recorder'],'center'}},'IconTransparency','off','InitLevel',3,'BlockName',struct('Token',{{'USB_FLIGHT_REC_BL1'}}),'MaskDescription',['Write input to the Flight Recorder. Recorded data can be referenced by the specified variable.'],'SampleTime',{{-1}})  RTIBlockParameters=struct('VarName',{{'powerConsumption_Ws','OFF',[]}},'DataType',{{'Single','OFF',[]}},'SampleTime',{{-1,'OFF',[]}},'TLCFileName',{{'rtiusbflightrecwrite','OFF',[]}})  RTISFcnParameters=struct('VarName','char','DataType','char','SampleTime','double','TLCFileName','char')  RTIBlockParaDefault=struct('VarName','Var1','DataType','Single','SampleTime',-1,'TLCFileName','rtiusbflightrecwrite')
      settings: SourceProductName=dSPACE RTI USB Flight Rec Blockset
  wires:
  Data Type Conversion/1 -> USB_FLIGHT_REC_BL1/1
  In1/1 -> Gain/1
  Gain/1 -> Data Type Conversion/1

== system DR18E_Testpult/Verarbeitung/Strom//SOC/powerRecorder ==
  In1 : Inport
  Data Type Conversion : DataTypeConversion
  Gain : Gain
  USB_FLIGHT_REC_BL1 : rtiusbflightreclib/USB_FLIGHT_REC_BL1  VarName=HV_power_W  DataType=Single  SampleTime=-1  TLCFileName=rtiusbflightrecwrite  Reserved1=[]  Reserved2=[]  Reserved3=[]  Reserved4=[]  DSProperties=struct('RTI',struct('Version',uint32(3),'BlockType',struct('isSLSource',uint8(0),'isSLSink',uint8(1),'isHWSource',uint8(0),'isHWSink',uint8(0),'isSetup',uint8(0),'isInline',uint8(1),'isNonInline',uint8(0),'isInterrupt',uint8(0),'isChannelwise',uint8(0)),'IOBoardType',{{'DSUSB','FLIGHTREC'}},'UnitType','FLIGHTREC','Identifier','WRITE','DialogType','SL','BlockSet','RTIUSBFLIGHTREC','SlaveProcessor','NONE'))  RTIBlockInterface=struct('InputPortsActive',1,'InputPortsWidth',int32(1),'InputPortsDataType',{{'SS_SINGLE'}},'BlockDisplay',{{['Write to\nUSB Flight Recorder'],'center'}},'IconTransparency','off','InitLevel',3,'BlockName',struct('Token',{{'USB_FLIGHT_REC_BL1'}}),'MaskDescription',['Write input to the Flight Recorder. Recorded data can be referenced by the specified variable.'],'SampleTime',{{-1}})  RTIBlockParameters=struct('VarName',{{'HV_power_W','OFF',[]}},'DataType',{{'Single','OFF',[]}},'SampleTime',{{-1,'OFF',[]}},'TLCFileName',{{'rtiusbflightrecwrite','OFF',[]}})  RTISFcnParameters=struct('VarName','char','DataType','char','SampleTime','double','TLCFileName','char')  RTIBlockParaDefault=struct('VarName','Var1','DataType','Single','SampleTime',-1,'TLCFileName','rtiusbflightrecwrite')
      settings: SourceProductName=dSPACE RTI USB Flight Rec Blockset
  wires:
  Data Type Conversion/1 -> USB_FLIGHT_REC_BL1/1
  In1/1 -> Gain/1
  Gain/1 -> Data Type Conversion/1

== system DR18E_Testpult/Verarbeitung/Temperaturregelung1/Detect Max Temp ==
  STK 1-5 : Inport
  STK 6-10 : Inport  Port=2
  Bus Selector : BusSelector  OutputSignals=STK1_Temp1-5.STK1_Temp1,STK1_Temp1-5.STK1_Temp2,STK1_Temp1-5.STK1_Temp3,STK1_Temp1-5.STK1_Temp4,STK1_Temp1-5.STK1_Temp5,STK2_Temp1-5.STK2_Temp1,STK2_Temp1-5.STK2_Temp2,STK2_Temp1-5.STK2_Temp3,STK2_Temp1-5.STK2_Temp4,STK2_Temp1-5.STK2_Temp5,STK3_Temp1-5.STK3_Temp1,STK3_Temp1-5.STK3_Temp2,STK3_Temp1-5.STK3_Temp3,STK3_Temp1-5.STK3_Temp4,STK3_Temp1-5.STK3_Temp5,STK4_Temp1-5.STK4_Temp1,STK4_Temp1-5.STK4_Temp2,STK4_Temp1-5.STK4_Temp3,STK4_Temp1-5.STK4_Temp4,STK4_Temp1-5.STK4_Temp5,STK5_Temp1-5.STK5_Temp1,STK5_Temp1-5.STK5_Temp2,STK5_Temp1-5.STK5_Temp3,STK5_Temp1-5.STK5_Temp4,STK5_Temp1-5.STK5_Temp5
  Bus Selector1 : BusSelector  OutputSignals=STK6_Temp1-5.STK6_Temp1,STK6_Temp1-5.STK6_Temp2,STK6_Temp1-5.STK6_Temp3,STK6_Temp1-5.STK6_Temp4,STK6_Temp1-5.STK6_Temp5,STK7_Temp1-5.STK7_Temp1,STK7_Temp1-5.STK7_Temp2,STK7_Temp1-5.STK7_Temp3,STK7_Temp1-5.STK7_Temp4,STK7_Temp1-5.STK7_Temp5,STK8_Temp1-5.STK8_Temp1,STK8_Temp1-5.STK8_Temp2,STK8_Temp1-5.STK8_Temp3,STK8_Temp1-5.STK8_Temp4,STK8_Temp1-5.STK8_Temp5,STK9_Temp1-5.STK9_Temp1,STK9_Temp1-5.STK9_Temp2,STK9_Temp1-5.STK9_Temp3,STK9_Temp1-5.STK9_Temp4,STK9_Temp1-5.STK9_Temp5,STK10_Temp1-5.STK10_Temp1,STK10_Temp1-5.STK10_Temp2,STK10_Temp1-5.STK10_Temp3,STK10_Temp1-5.STK10_Temp4,STK10_Temp1-5.STK10_Temp5
  MinMax : MinMax  Function=max  Inputs=25
  MinMax1 : MinMax  Function=max  Inputs=25
  MinMax2 : MinMax  Function=max  Inputs=2
  HV Battery Max Temp : Outport
  wires:
  STK 1-5/1 -> Bus Selector/1
  Bus Selector/25 -> MinMax/25  "<STK5_Temp5>"
  Bus Selector/24 -> MinMax/24  "<STK5_Temp4>"
  Bus Selector/23 -> MinMax/23  "<STK5_Temp3>"
  Bus Selector/22 -> MinMax/22  "<STK5_Temp2>"
  Bus Selector/21 -> MinMax/21  "<STK5_Temp1>"
  Bus Selector/20 -> MinMax/20  "<STK4_Temp5>"
  Bus Selector/19 -> MinMax/19  "<STK4_Temp4>"
  Bus Selector/18 -> MinMax/18  "<STK4_Temp3>"
  Bus Selector/17 -> MinMax/17  "<STK4_Temp2>"
  Bus Selector/16 -> MinMax/16  "<STK4_Temp1>"
  Bus Selector/15 -> MinMax/15  "<STK3_Temp5>"
  Bus Selector/14 -> MinMax/14  "<STK3_Temp4>"
  Bus Selector/13 -> MinMax/13  "<STK3_Temp3>"
  Bus Selector/12 -> MinMax/12  "<STK3_Temp2>"
  Bus Selector/11 -> MinMax/11  "<STK3_Temp1>"
  Bus Selector/10 -> MinMax/10  "<STK2_Temp5>"
  Bus Selector/9 -> MinMax/9  "<STK2_Temp4>"
  Bus Selector/8 -> MinMax/8  "<STK2_Temp3>"
  Bus Selector/7 -> MinMax/7  "<STK2_Temp2>"
  Bus Selector/6 -> MinMax/6  "<STK2_Temp1>"
  Bus Selector/5 -> MinMax/5  "<STK1_Temp5>"
  Bus Selector/4 -> MinMax/4  "<STK1_Temp4>"
  Bus Selector/3 -> MinMax/3  "<STK1_Temp3>"
  Bus Selector/2 -> MinMax/2  "<STK1_Temp2>"
  Bus Selector/1 -> MinMax/1  "<STK1_Temp1>"
  MinMax2/1 -> HV Battery Max Temp/1
  MinMax/1 -> MinMax2/1
  Bus Selector1/20 -> MinMax1/20  "<STK9_Temp5>"
  Bus Selector1/21 -> MinMax1/21  "<STK10_Temp1>"
  Bus Selector1/23 -> MinMax1/23  "<STK10_Temp3>"
  Bus Selector1/19 -> MinMax1/19  "<STK9_Temp4>"
  Bus Selector1/22 -> MinMax1/22  "<STK10_Temp2>"
  Bus Selector1/24 -> MinMax1/24  "<STK10_Temp4>"
  MinMax1/1 -> MinMax2/2
  STK 6-10/1 -> Bus Selector1/1
  Bus Selector1/1 -> MinMax1/1  "<STK6_Temp1>"
  Bus Selector1/2 -> MinMax1/2  "<STK6_Temp2>"
  Bus Selector1/3 -> MinMax1/3  "<STK6_Temp3>"
  Bus Selector1/4 -> MinMax1/4  "<STK6_Temp4>"
  Bus Selector1/5 -> MinMax1/5  "<STK6_Temp5>"
  Bus Selector1/6 -> MinMax1/6  "<STK7_Temp1>"
  Bus Selector1/7 -> MinMax1/7  "<STK7_Temp2>"
  Bus Selector1/8 -> MinMax1/8  "<STK7_Temp3>"
  Bus Selector1/9 -> MinMax1/9  "<STK7_Temp4>"
  Bus Selector1/10 -> MinMax1/10  "<STK7_Temp5>"
  Bus Selector1/11 -> MinMax1/11  "<STK8_Temp1>"
  Bus Selector1/12 -> MinMax1/12  "<STK8_Temp2>"
  Bus Selector1/13 -> MinMax1/13  "<STK8_Temp3>"
  Bus Selector1/14 -> MinMax1/14  "<STK8_Temp4>"
  Bus Selector1/15 -> MinMax1/15  "<STK8_Temp5>"
  Bus Selector1/16 -> MinMax1/16  "<STK9_Temp1>"
  Bus Selector1/17 -> MinMax1/17  "<STK9_Temp2>"
  Bus Selector1/18 -> MinMax1/18  "<STK9_Temp3>"
  Bus Selector1/25 -> MinMax1/25  "<STK10_Temp5>"

== system DR18E_Testpult/Verarbeitung/Temperaturregelung1/ModeSelect ==
  Man/Aut Pulse : Inport
  Value Man : Inport  Port=2
  Value Aut : Inport  Port=3
  Constant : Constant  OutDataTypeStr=Inherit: Inherit via back propagation
  Data Type Conversion : DataTypeConversion  OutDataTypeStr=boolean
  J-K Flip-Flop : simulink_extras/Flip Flops/J-K Flip-Flop  initial_condition=0
      settings: SourceProductName=Simulink
  Switch : Switch  Criteria=u2 > Threshold
  Value : Outport
  wires:
  Value Man/1 -> Switch/1
  Value Aut/1 -> Switch/3
  Switch/1 -> Value/1
  Constant/1 -> J-K Flip-Flop/3, J-K Flip-Flop/1
  Man/Aut Pulse/1 -> Data Type Conversion/1
  J-K Flip-Flop/1 -> Switch/2  "Man/!Aut"
  Data Type Conversion/1 -> J-K Flip-Flop/2
